simulink model "AircraftDynamicsModel"  (R2024b)
settings: Solver=ode45  StartTime=0.0  StopTime=20  RelTol=1e-3
model workspace (MAT data in the model file):
  g = 1
settings Model: Creator=Evan Peres  LastModifiedBy=Evan Peres

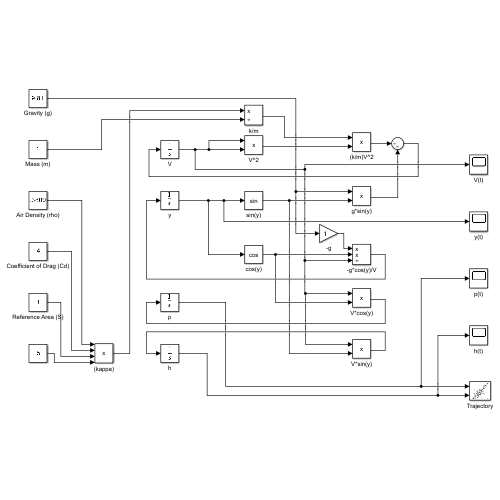
[thumbnail: Simulink's stored preview of the top-level diagram]
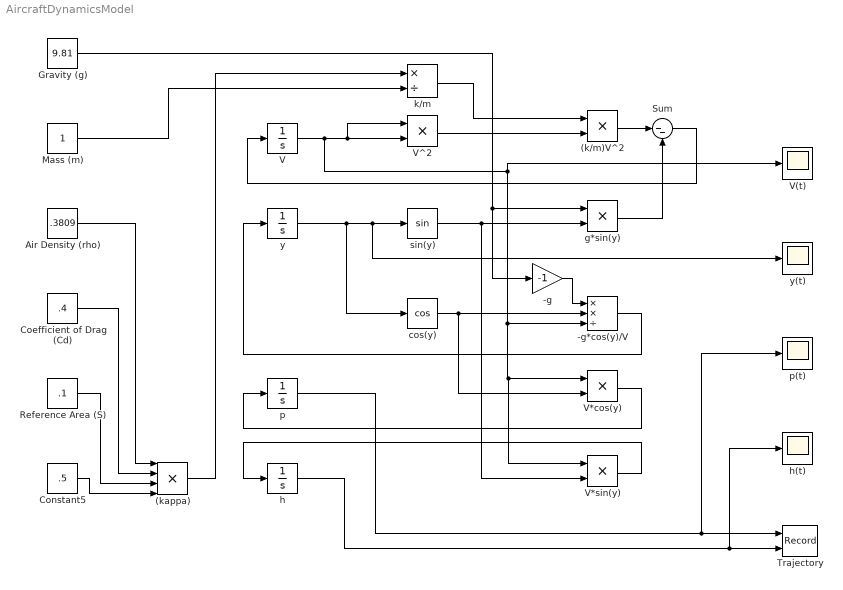
== system AircraftDynamicsModel ==
  (k/m)V^2 : Product
  (kappa) : Product  Inputs=4
  -g : Gain  Gain=-1
  -g*cos(y)/V : Product  Inputs=**/
  Air Density (rho) : Constant  Value=.3809
  Coefficient of Drag (Cd) : Constant  Value=.4
  Constant5 : Constant  Value=.5
  Gravity (g) : Constant  Value=9.81
  Mass (m) : Constant
  Reference Area (S) : Constant  Value=.1
  Sum : Sum  Inputs=|--
  Trajectory : Record  FileSettingsInternal="{\"entries\":[{\"content\":{\"excelSettings\":{\"content\":{},\"type\":\"Streamout.ExcelSettings\"}},\"type\":\"Streamout.FileSettingStorage\",\"uuid\":\"\"}],\"packageUris\":[\"http:\\/\\/schema.mathworks.com\\/mf0\\/streamout_blocks\\/R2020a\"],\"version\":\"1.0\"}"  Layout=[1 1]  SignalsInternal="{\"entries\":[{\"content\":{\"signals\":[{\"content\":{\"blockPath\":[],\"dimensions\":[1],\"domain\":\"\",\"lineColor\":\"#64d413\",\"lineWidth\":2,\"plots\":[ 1 ],\"port\":1,\"sid\":[\"\"],\"signalID\":1,\"signalName\":\"p\"},\"type\":\"RecordBlkView.Signal\",\"uuid\":\"\"},{\"content\":{\"blockPath\":[],\"dimensions\":[1],\"domain\":\"\",\"lineColor\":\"#139fff\",\"plots\":[ 1 ],\"port\":2,\"sid\":[\"\"],\"signalID\":2,\"signalName\":\"h\"},\"type\":\"RecordBlkView.Signal\",\"uuid\":\"\"}]},\"type\":\"RecordBlkView.InputSignals\",\"uuid\":\"\"}],\"packageUris\":[\"http:\\/\\/schema.mathworks.com\\/mf0\\/streamout_blocks\\/R2020a\"],\"version\":\"1.0\"}"  VisualizationBindings="{\"xyplotplugin\":{\"info\":[{\"series\":[{\"bindingParametersList\":[{\"parameter\":\"X-Axis\",\"signalID\":1,\"signalName\":\"p\"},{\"parameter\":\"Y-Axis\",\"signalID\":2,\"signalName\":\"h\"},{\"parameter\":\"X-Axis\",\"signalID\":1,\"signalName\":\"p\"},{\"parameter\":\"Y-Axis\",\"signalID\":2,\"signalName\":\"h\"}],\"seriesID\":0}],\"subplotID\":1}]}}"  CompatibilityTag=XY
  V : Integrator  InitialCondition=10
  V(t) : Scope
  V*cos(y) : Product
  V*sin(y) : Product
  V^2 : Product
  cos(y) : Trigonometry  Operator=cos
  g*sin(y) : Product
  h : Integrator  InitialCondition=100
  h(t) : Scope
  k/m : Product  Inputs=*/
  p : Integrator
  p(t) : Scope
  sin(y) : Trigonometry
  y : Integrator  InitialCondition=pi/4
  y(t) : Scope
  wires:
  Constant5/1 -> (kappa)/4
  Air Density (rho)/1 -> (kappa)/1
  Coefficient of Drag (Cd)/1 -> (kappa)/2
  Reference Area (S)/1 -> (kappa)/3
  sin(y)/1 -> V*sin(y)/2, g*sin(y)/2
  Gravity (g)/1 -> -g/1, g*sin(y)/1
  y/1 -> cos(y)/1, y(t)/1, sin(y)/1
  V/1 -> V*sin(y)/1, V*cos(y)/1, -g*cos(y)/V/3, V(t)/1, V^2/1, V^2/2
  (kappa)/1 -> k/m/1
  k/m/1 -> (k/m)V^2/1
  Mass (m)/1 -> k/m/2
  V^2/1 -> (k/m)V^2/2
  (k/m)V^2/1 -> Sum/1
  g*sin(y)/1 -> Sum/2
  Sum/1 -> V/1
  -g/1 -> -g*cos(y)/V/1
  cos(y)/1 -> V*cos(y)/2, -g*cos(y)/V/2
  -g*cos(y)/V/1 -> y/1
  V*cos(y)/1 -> p/1
  V*sin(y)/1 -> h/1
  h/1 -> Trajectory/2, h(t)/1
  p/1 -> Trajectory/1, p(t)/1
